simulink model "LinearIPS_StepInput_Final"  (R2022a)
settings: Solver=FixedStepAuto  StartTime=0.0  StopTime=2  FixedStep=T  RelTol=1e-3
undefined symbols (not defined in the file): DAS6036, G, Measurement_Computing, PCI, QUAD04, T
libraries: sldrtlib x2
settings Model: SimulationMode=external  ExtModeTrigDuration=100000  Creator=Controls Lab  LastModifiedBy=Mechatronics
settings SolverCC: AlgebraicLoopSolver=TrustRegion
settings DebuggingCC: UnconnectedInputMsg=warning  UnconnectedOutputMsg=warning  UnconnectedLineMsg=warning  SFMachineParentedDataDiag=warning
settings HardwareCC: ProdBitPerLong=64  ProdHWDeviceType=Intel->x86-64 (Linux 64)
settings SFSimCC: CustomCodeUndefinedFunction=UseInterfaceOnly
settings RTWCC: Description=Simulink Desktop Real-Time  SystemTargetFile=sldrt.tlc  TemplateMakefile=sldrt.tmf  RTWCompilerOptimization=on  DLArmComputeVersion=19.05
settings CodeAppCC: MaxIdLength=95
settings SimulinkDesktopRealTimeCC: TargetLibSuffix=_sldrt.a  TargetPreCompLibLocation=C:\Program Files\MATLAB\R2022a\toolbox\sldrt\lib\win64

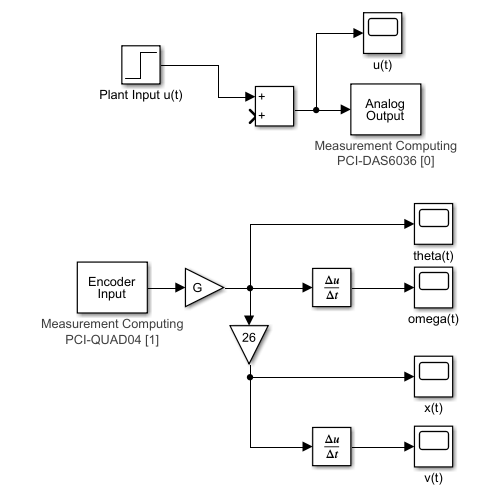
[thumbnail: Simulink's stored preview of the top-level diagram]
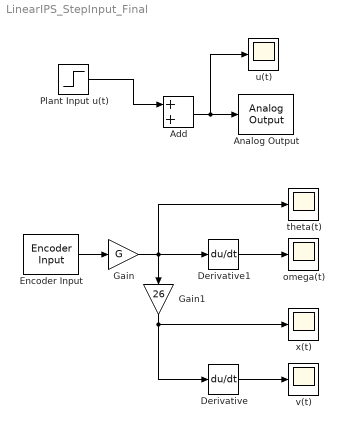
== system LinearIPS_StepInput_Final ==
  Add : Sum
  Analog Output : sldrtlib/Analog Output  SampleTime=T  MaxMissedTicks=10  ShowMissedTicks=off  YieldWhenWaiting=off  DrvName=Measurement_Computing/PCI-DAS6036  DrvAddress=0  DrvOptions=[0 0 0]  Channels=1  RangeMode=1  VoltRange=1  InitialValue=0  FinalValue=0
      settings: AttributesFormatString=Measurement Computing\nPCI-DAS6036 [0]
  Derivative : Derivative
  Derivative1 : Derivative
  Encoder Input : sldrtlib/Encoder Input  SampleTime=T  MaxMissedTicks=10  ShowMissedTicks=off  YieldWhenWaiting=off  DrvName=Measurement_Computing/PCI-QUAD04  DrvAddress=1  DrvOptions=zeros(1,0)  Channels=2  QuadMode=3  IndexPulse=3  InputFilter=Inf  DataType=1
      settings: AttributesFormatString=Measurement Computing\nPCI-QUAD04 [1]
  Gain : Gain  Gain=G
  Gain1 : Gain  Gain=26
  Plant Input u(t) : Step  Time=0  After=0.75  SampleTime=T
  omega(t) : Scope
  theta(t) : Scope
  u(t) : Scope
  v(t) : Scope
  x(t) : Scope
  wires:
  Encoder Input/1 -> Gain/1
  Gain/1 -> Derivative1/1, theta(t)/1, Gain1/1
  Derivative1/1 -> omega(t)/1
  Gain1/1 -> Derivative/1, x(t)/1
  Derivative/1 -> v(t)/1
  Add/1 -> u(t)/1, Analog Output/1
  Plant Input u(t)/1 -> Add/1
